simulink model "V4_Modell_komplett"  (R2022b)
settings: Solver=ode3  StartTime=0.0  StopTime=Zeit(end)  FixedStep=1e-5  RelTol=1e-3
values from neighbouring files (symbols this model uses):
  k_M = C_Phi    (= 42.43)    [V4_Parameter_Parameter_komplett_te.m]    (also in V4_Parameter_Wagen_Te.m = 0.04243; V4_Parameter_komplett.m = 0.04243)
  r_ZR = 0.021    [V4_Parameter_Parameter_komplett_te.m]    (also in V4_Parameter_Wagen_Te.m; V4_Parameter_komplett.m)
settings Model: Creator=fstic  LastModifiedBy=JSCHB

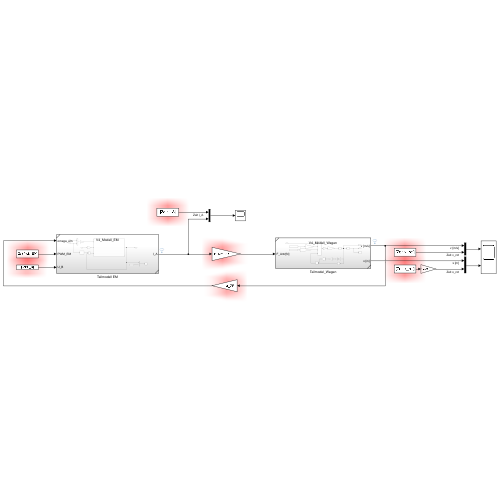
[thumbnail: Simulink's stored preview of the top-level diagram]
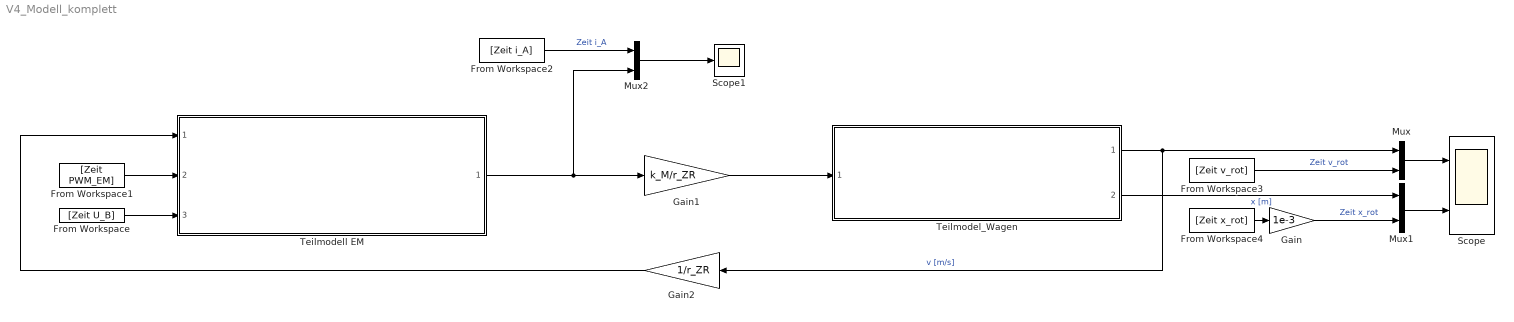
== system V4_Modell_komplett ==
  From Workspace : FromWorkspace  VariableName=[Zeit U_B]
  From Workspace1 : FromWorkspace  VariableName=[Zeit PWM_EM]
  From Workspace2 : FromWorkspace  VariableName=[Zeit i_A]
  From Workspace3 : FromWorkspace  VariableName=[Zeit v_rot]
  From Workspace4 : FromWorkspace  VariableName=[Zeit x_rot]
  Gain : Gain  Gain=1e-3
  Gain1 : Gain  Gain=k_M/r_ZR
  Gain2 : Gain  Gain=1/r_ZR
  Mux : Mux  Inputs=2
  Mux1 : Mux  Inputs=2
  Mux2 : Mux  Inputs=2
  Scope : Scope  NumInputPorts=2
  Scope1 : Scope
  Teilmodel_Wagen : Subsystem  ReferencedSubsystem=V4_Modell_Wagen
  Teilmodell EM : Subsystem  ReferencedSubsystem=V4_Modell_EM
  wires:
  Mux/1 -> Scope/1
  Teilmodel_Wagen/1 -> Gain2/1, Mux/1  "v [m/s]"
  Mux1/1 -> Scope/2
  Teilmodel_Wagen/2 -> Mux1/1  "x [m]"
  Gain/1 -> Mux1/2  "Zeit x_rot"
  Teilmodell EM/1 -> Mux2/2, Gain1/1
  Gain1/1 -> Teilmodel_Wagen/1
  Mux2/1 -> Scope1/1
  From Workspace2/1 -> Mux2/1  "Zeit i_A"
  From Workspace3/1 -> Mux/2  "Zeit v_rot"
  From Workspace4/1 -> Gain/1
  Gain2/1 -> Teilmodell EM/1
  From Workspace1/1 -> Teilmodell EM/2
  From Workspace/1 -> Teilmodell EM/3
